simulink model "sim_env"  (R2023b)
settings: Solver=VariableStepAuto  StartTime=0.0  StopTime=10.0  RelTol=1e-3
undefined symbols (not defined in the file): mass
libraries: shared6dof x1, aerolibanim x1, robotcorelib x1
settings Model: Creator=Zian Liu  LastModifiedBy=Zian Liu

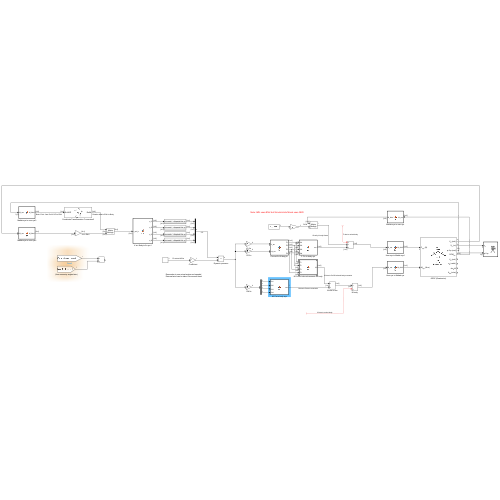
[thumbnail: Simulink's stored preview of the top-level diagram]
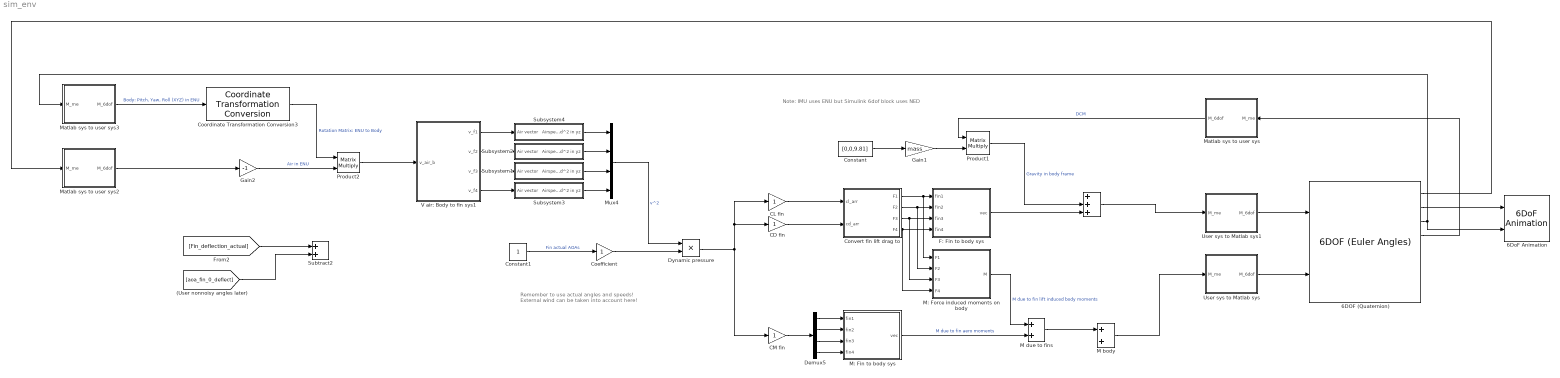
== system sim_env ==
  note: Note: IMU uses ENU but Simulink 6dof block uses NED
  note: Remember to use actual angles and speeds!
      | External wind can be taken into account here!
  " " : Sum  Inputs=+++
  6DOF (Quaternion) : shared6dof/6DOF (Euler Angles)  units=Metric (MKS)  mtype=Fixed  rep=Quaternion  xme_0=[0 0 0]  Vm_0=[0 0 0]  eul_0=[0 0 0]  pm_0=[0 0 0]  mass_0=1.0  mass_e=0.5  mass_f=2.0  inertia=eye(3)  inertia_e=eye(3)  inertia_f=2*eye(3)  k_quat=1.0  vre_flag=on  abi_flag=off  aMode=0  xme_statename=''  Vm_statename=''  eul_statename=''  quat_statename={'qr', 'qi', 'qj','qk'}  pm_statename=''  mass_statename=''
      settings: LibrarySourceBlock=aerolib6dof2/6DOF (Quaternion)
  6DoF Animation : aerolibanim/6DoF Animation  u1=[0 4000 -2000 2000 -5000 -3000]  u2=0.1  u3=1.0  u4=[4000 0 -5000]  u5=Fixed position  u6=[2000 500 -3150]  u7=10  u8=on
  CD fin : Gain
  CL fin : Gain
  CM fin : Gain
  Coefficient : Gain
  Constant : Constant  Value=[0,0,9.81]
  Constant1 : Constant
  "Convert fin lift drag to " : MATLAB Function  TreatAsAtomicUnit=on
  Coordinate Transformation Conversion3 : robotcorelib/Coordinate Transformation Conversion  InputRepresentation=Euler Angles  InputEulerSequence=XYZ  ShowTrVecInputPort=on  OutputRepresentation=Rotation Matrix  OutputEulerSequence=XYZ  ShowTrVecOutputPort=on  SimulateUsing=Interpreted execution
      settings: LibrarySourceBlock=uavutilslib/Coordinate Transformation Conversion
  Demux5 : Demux
  Dynamic pressure : Product
  F: Fin to body sys : MATLAB Function  TreatAsAtomicUnit=on
  Gain1 : Gain  Gain=mass
  Gain2 : Gain  Gain=-1
  M body : Sum
  M due to fins : Sum
  M: Fin to body sys : MATLAB Function  TreatAsAtomicUnit=on
  M: Force induced moments on body : MATLAB Function  TreatAsAtomicUnit=on
  Matlab sys to user sys : MATLAB Function  TreatAsAtomicUnit=on
  Matlab sys to user sys2 : MATLAB Function  TreatAsAtomicUnit=on
  Matlab sys to user sys3 : MATLAB Function  TreatAsAtomicUnit=on
  Mux4 : Mux
  Product1 : Product  Multiplication=Matrix(*)
  Product2 : Product  Multiplication=Matrix(*)
  Subsystem1 : Subsystem
  Subsystem2 : Subsystem
  Subsystem3 : Subsystem
  Subsystem4 : Subsystem
  Subtract2 : Sum
  User sys to Matlab sys : MATLAB Function  TreatAsAtomicUnit=on
  User sys to Matlab sys1 : MATLAB Function  TreatAsAtomicUnit=on
  V air: Body to fin sys1 : MATLAB Function  TreatAsAtomicUnit=on
  wires:
  Matlab sys to user sys2/1(M_6dof) -> Gain2/1
  Gain2/1 -> Product2/2  "Air in ENU"
  Subsystem1/1(Airspeed^2 in yz) -> Mux4/3
  Coordinate Transformation Conversion3/1 -> Product2/1  "Rotation Matrix: ENU to Body"
  Subsystem2/1(Airspeed^2 in yz) -> Mux4/2
  Coefficient/1 -> Dynamic pressure/2
  V air: Body to fin sys1/2(v_f2) -> Subsystem2/1(Air vector)
  V air: Body to fin sys1/4(v_f4) -> Subsystem3/1(Air vector)
  Subsystem4/1(Airspeed^2 in yz) -> Mux4/1
  V air: Body to fin sys1/1(v_f1) -> Subsystem4/1(Air vector)
  Matlab sys to user sys/1(M_6dof) -> Product1/1  "DCM"
  Constant1/1 -> Coefficient/1  "Fin actual AOAs"
  [aoa_fin_0_deflect] -> Subtract2/2
  Matlab sys to user sys3/1(M_6dof) -> Coordinate Transformation Conversion3/1  "Body: Pitch, Yaw, Roll (XYZ) in ENU"
  F: Fin to body sys/1(vec) -> " "/3
  Subsystem3/1(Airspeed^2 in yz) -> Mux4/4
  Gain1/1 -> Product1/2
  M due to fins/1 -> M body/1
  " "/1 -> User sys to Matlab sys1/1(M_me)
  "Convert fin lift drag to "/4(F4) -> M: Force induced moments on body/4(F4), F: Fin to body sys/4(fin4)
  M: Force induced moments on body/1(M) -> M due to fins/1  "M due to fin lift induced body moments"
  User sys to Matlab sys/1(M_6dof) -> 6DOF (Quaternion)/2
  Constant/1 -> Gain1/1
  CM fin/1 -> Demux5/1
  M body/1 -> User sys to Matlab sys/1(M_me)
  V air: Body to fin sys1/3(v_f3) -> Subsystem1/1(Air vector)
  ? -> M body/2  "M due to rocket body"
  Demux5/2 -> M: Fin to body sys/2(fin2)
  "Convert fin lift drag to "/2(F2) -> M: Force induced moments on body/2(F2), F: Fin to body sys/2(fin2)
  "Convert fin lift drag to "/1(F1) -> M: Force induced moments on body/1(F1), F: Fin to body sys/1(fin1)
  "Convert fin lift drag to "/3(F3) -> M: Force induced moments on body/3(F3), F: Fin to body sys/3(fin3)
  Demux5/3 -> M: Fin to body sys/3(fin3)
  [Fin_deflection_actual] -> Subtract2/1
  ? -> " "/1  "F due to rocket body"
  Demux5/1 -> M: Fin to body sys/1(fin1)
  Demux5/4 -> M: Fin to body sys/4(fin4)
  CL fin/1 -> "Convert fin lift drag to "/1(cl_arr)
  M: Fin to body sys/1(vec) -> M due to fins/2  "M due to fin aero moments"
  CD fin/1 -> "Convert fin lift drag to "/2(cd_arr)
  User sys to Matlab sys1/1(M_6dof) -> 6DOF (Quaternion)/1
  Dynamic pressure/1 -> CL fin/1, CD fin/1, CM fin/1
  Mux4/1 -> Dynamic pressure/1  "v^2"
  Product1/1 -> " "/2  "Gravity in body frame"
  6DOF (Quaternion)/4 -> Matlab sys to user sys/1(M_me)
  6DOF (Quaternion)/1 -> Matlab sys to user sys2/1(M_me)
  6DOF (Quaternion)/3 -> 6DoF Animation/2, Matlab sys to user sys3/1(M_me)
  6DOF (Quaternion)/2 -> 6DoF Animation/1
  Product2/1 -> V air: Body to fin sys1/1(v_air_b)

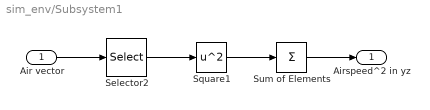
== system sim_env/Subsystem1 ==
  Air vector : Inport
  Selector2 : Selector  InputPortWidth=3  IndexOptions=Index vector (dialog)  Indices=[2 3]  OutputSizes=1
  Square1 : Math  Operator=square
  Sum of Elements : Sum  Inputs=+
  Airspeed^2 in yz : Outport
  wires:
  Square1/1 -> Sum of Elements/1
  Selector2/1 -> Square1/1
  Sum of Elements/1 -> Airspeed^2 in yz/1
  Air vector/1 -> Selector2/1

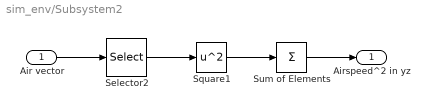
== system sim_env/Subsystem2 ==
  Air vector : Inport
  Selector2 : Selector  InputPortWidth=3  IndexOptions=Index vector (dialog)  Indices=[2 3]  OutputSizes=1
  Square1 : Math  Operator=square
  Sum of Elements : Sum  Inputs=+
  Airspeed^2 in yz : Outport
  wires:
  Square1/1 -> Sum of Elements/1
  Selector2/1 -> Square1/1
  Sum of Elements/1 -> Airspeed^2 in yz/1
  Air vector/1 -> Selector2/1

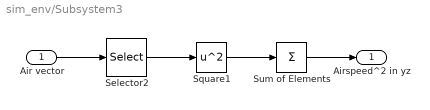
== system sim_env/Subsystem3 ==
  Air vector : Inport
  Selector2 : Selector  InputPortWidth=3  IndexOptions=Index vector (dialog)  Indices=[2 3]  OutputSizes=1
  Square1 : Math  Operator=square
  Sum of Elements : Sum  Inputs=+
  Airspeed^2 in yz : Outport
  wires:
  Square1/1 -> Sum of Elements/1
  Selector2/1 -> Square1/1
  Sum of Elements/1 -> Airspeed^2 in yz/1
  Air vector/1 -> Selector2/1

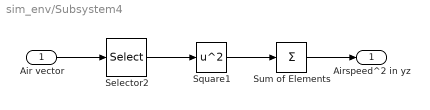
== system sim_env/Subsystem4 ==
  Air vector : Inport
  Selector2 : Selector  InputPortWidth=3  IndexOptions=Index vector (dialog)  Indices=[2 3]  OutputSizes=1
  Square1 : Math  Operator=square
  Sum of Elements : Sum  Inputs=+
  Airspeed^2 in yz : Outport
  wires:
  Square1/1 -> Sum of Elements/1
  Selector2/1 -> Square1/1
  Sum of Elements/1 -> Airspeed^2 in yz/1
  Air vector/1 -> Selector2/1

== matlab function sim_env/F: Fin to body sys ==
  data: fin1 input; vec output; fin2 input; fin3 input; fin4 input
function vec = fcn(fin1, fin2, fin3, fin4)
vx = fin1(1) - fin2(2) - fin3(1) + fin4(2);
vy = fin1(2) + fin2(1) - fin3(2) - fin4(1);
vz = fin1(3) + fin2(3) + fin3(3) + fin4(3);

vec = [vx, vy, vz];

== matlab function sim_env/M: Fin to body sys ==
  data: fin1 input; vec output; fin2 input; fin3 input; fin4 input
function vec = fcn(fin1, fin2, fin3, fin4)
vx = fin1(1) - fin2(2) - fin3(1) + fin4(2);
vy = fin1(2) + fin2(1) - fin3(2) - fin4(1);
vz = fin1(3) + fin2(3) + fin3(3) + fin4(3);

vec = [vx, vy, vz];

== matlab function sim_env/M: Force induced moments on body ==
  data: F1 input; M output; F2 input; F3 input; F4 input
function M = fcn(F1, F2, F3, F4)
r_arm_moment = 1;
l_arm_moment = 1;
r1 = [r_arm_moment, 0, -l_arm_moment];
r2 = [0, r_arm_moment, -l_arm_moment];
r3 = [-r_arm_moment, 0, -l_arm_moment];
r4 = [0, -r_arm_moment, -l_arm_moment];
M = cross(r1, F1) + cross(r2, F2) + cross(r3, F3) + cross(r4, F4);

== matlab function sim_env/Convert fin lift drag to  ==
  data: cl_arr input; F1 output; cd_arr input; F2 output; F3 output; F4 output
function [F1, F2, F3, F4]= fcn(cl_arr, cd_arr)
F1 = [0, cl_arr(1), -cd_arr(1)];
F2 = [0, cl_arr(2), -cd_arr(2)];
F3 = [0, cl_arr(3), -cd_arr(3)];
F4 = [0, cl_arr(4), -cd_arr(4)];

== matlab function sim_env/User sys to Matlab sys ==
  data: M_me input; M_6dof output
function M_6dof = fcn(M_me)
M_6dof = [M_me(3), M_me(1), M_me(2)];

== matlab function sim_env/User sys to Matlab sys1 ==
  data: M_me input; M_6dof output
function M_6dof = fcn(M_me)
M_6dof = [M_me(3), M_me(1), M_me(2)];

== matlab function sim_env/V air: Body to fin sys1 ==
  data: v_air_b input; v_f1 output; v_f2 output; v_f3 output; v_f4 output
function [v_f1, v_f2, v_f3, v_f4]= fcn(v_air_b)
vx = v_air_b(1);
vy = v_air_b(2);
vz = v_air_b(3);

v_f1 = [vx, vy, vz];
v_f2 = [vy, -vx, vz];
v_f3 = [-vx, -vy, vz];
v_f4 = [-vy, vx, vz];

== matlab function sim_env/Matlab sys to user sys ==
  data: M_me input; M_6dof output
function M_6dof = fcn(M_me)
M_6dof = [M_me(3), M_me(1), M_me(2)];

== matlab function sim_env/Matlab sys to user sys2 ==
  data: M_me input; M_6dof output
function M_6dof = fcn(M_me)
M_6dof = [M_me(3); M_me(1); M_me(2)];

== matlab function sim_env/Matlab sys to user sys3 ==
  data: M_me input; M_6dof output
function M_6dof = fcn(M_me)
M_6dof = [M_me(3), M_me(1), M_me(2)];
